simulink model "CrCtl_StTrans"  (R2016b)
settings: configuration reference "CodeGenConfigSet" (kept outside this file)
values from neighbouring files (symbols this model uses):
  CrCtl_swtAllwSetDrngOvrd_C = Calibration.Parameter    [init_CrCtl_StTrans.m]
  CrCtl_swtWESDem_C = Calibration.Parameter    [init_CrCtl_StTrans.m]
  CrCtl_tiEnaAftShOff_C = Calibration.Parameter    [init_CrCtl_StTrans.m]
  CrCtl_vAcclLoLim_C = Calibration.Parameter    [init_CrCtl_StTrans.m]
  CrCtl_vAcclUpLim_C = Calibration.Parameter    [init_CrCtl_StTrans.m]
  CrCtl_vDeclLoLim_C = Calibration.Parameter    [init_CrCtl_StTrans.m]
  CrCtl_vDeclUpLim_C = Calibration.Parameter    [init_CrCtl_StTrans.m]
  CrCtl_vEnaAftShOff_C = Calibration.Parameter    [init_CrCtl_StTrans.m]
  CrCtl_vMinAct_C = Calibration.Parameter    [init_CrCtl_StTrans.m]
  MoFCCtl_vCrCtlMin_C = Calibration.Parameter    [init_CrCtl_StTrans.m]
  VEL_ZERO = fi(0,VehSpeed_km_h)    [init_CrCtl_StTrans.m]
undefined symbols (not defined in the file or in its folder): CrCtl_stLck_conv, CrCtl_stOpFunc_conv, CrCtl_stShOff_conv, CrCtl_stSub_conv, CrCtl_StTrans_DT, CrCUI_BttnState_conv, CruiseCtl_State_conv, WESDem_State_conv
libraries: CXLib x4
settings Model: Creator=guanxiaoxing  LastModifiedBy=guanxiaoxing
settings ConfigSetRef: SourceLocation=Base Workspace

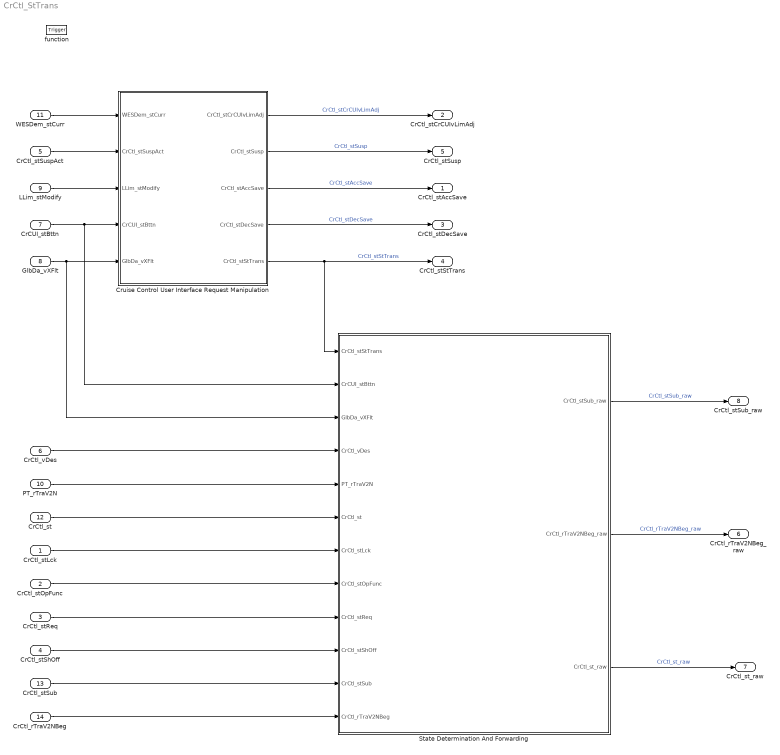
== system CrCtl_StTrans ==
  CrCtl_stLck : Inport  Description=Cruise Control lock Status  OutDataTypeStr=Enum: CrCtl_stLck_conv
  CrCtl_stOpFunc : Inport  Description=state of cruise control operation functionality  Port=2  OutDataTypeStr=Enum: CrCtl_stOpFunc_conv
  CrCtl_stReq : Inport  Description=Cruise control is active  Port=3  OutMin=0  OutMax=1  OutDataTypeStr=boolean
  CrCtl_stShOff : Inport  Description=cruise control shut-off requirement  Port=4  OutDataTypeStr=Enum: CrCtl_stShOff_conv
  CrCtl_stSuspAct : Inport  Description=Cruise Control suspend mode active Status  Port=5  OutMin=0  OutMax=1  OutDataTypeStr=boolean
  CrCtl_vDes : Inport  Tag=km/h  Description=Cruise Control desired set point speed  Port=6  OutMin=0  OutMax=250  OutDataTypeStr=VehSpeed_km_h
  CrCUI_stBttn : Inport  Description=Application parameter for status button information  Port=7  OutDataTypeStr=Enum: CrCUI_BttnState_conv
  GlbDa_vXFlt : Inport  Tag=km/h  Description=Vehicle velocity filtered  Port=8  OutMin=0  OutMax=250  OutDataTypeStr=VehSpeed_km_h
  LLim_stModify : Inport  Description=Application parameter for Status for changing adjustable vehicle speed limit  Port=9  OutMin=0  OutMax=1  OutDataTypeStr=boolean
  PT_rTraV2N : Inport  Tag=km/h/rpm  Description=Quotient of velocity and engine speed  Port=10  OutMin=-0.32768  OutMax=0.32767  OutDataTypeStr=Tra_V2N_km_h_rpm
  WESDem_stCurr : Inport  Description=Status of the working engine Speed Control  Port=11  OutDataTypeStr=Enum: WESDem_State_conv
  CrCtl_st : Inport  Description=Application parameter for Cruise Control state  Port=12  OutDataTypeStr=Enum: CruiseCtl_State_conv
  CrCtl_stSub : Inport  Description=Cruise control sub mode  Port=13  OutDataTypeStr=Enum: CrCtl_stSub_conv
  CrCtl_rTraV2NBeg : Inport  Tag=km/h/rpm  Description=V/N ratio at activation of cruise control  Port=14  OutMin=-0.32768  OutMax=0.32767  OutDataTypeStr=Tra_V2N_km_h_rpm
  function : TriggerPort  TriggerType=function-call  VariantControl=Variant
  Cruise Control User Interface Request Manipulation : Subsystem
  State Determination And Forwarding : Subsystem
  CrCtl_stAccSave : Outport  Description=|  OutDataTypeStr=Enum: CrCUI_BttnState_conv
      | Last CrCui state below the minimum speed to
      | activate
  CrCtl_stCrCUIvLimAdj : Outport  Description=CrCui Status of Limitation adjustment by Cruise control  Port=2  OutDataTypeStr=Enum: CrCUI_BttnState_conv
  CrCtl_stDecSave : Outport  Description=|  Port=3  OutDataTypeStr=Enum: CrCUI_BttnState_conv
      | Last CrCui state above the minimum speed to
      | activate
  CrCtl_stStTrans : Outport  Description=State transition demand to the state machine of cruise control  Port=4  OutDataTypeStr=Enum: CrCUI_BttnState_conv
  CrCtl_stSusp : Outport  Description=Status of Cruise control suspend mode  Port=5  OutDataTypeStr=Enum: CrCUI_BttnState_conv
  CrCtl_rTraV2NBeg_raw : Outport  Tag=km/h/rpm  Description=V/N ratio at activation of cruise control  Port=6  OutMin=-0.32768  OutMax=0.32767  OutDataTypeStr=Tra_V2N_km_h_rpm
  CrCtl_st_raw : Outport  Description=Application parameter for Cruise Control state  Port=7  OutDataTypeStr=Enum: CruiseCtl_State_conv
  CrCtl_stSub_raw : Outport  Description=Cruise control sub mode  Port=8  OutDataTypeStr=Enum: CrCtl_stSub_conv
  wires:
  WESDem_stCurr/1 -> Cruise Control User Interface Request Manipulation/1(WESDem_stCurr)
  CrCtl_stSuspAct/1 -> Cruise Control User Interface Request Manipulation/2(CrCtl_stSuspAct)
  LLim_stModify/1 -> Cruise Control User Interface Request Manipulation/3(LLim_stModify)
  CrCUI_stBttn/1 -> Cruise Control User Interface Request Manipulation/4(CrCUI_stBttn), State Determination And Forwarding/2(CrCUI_stBttn)
  GlbDa_vXFlt/1 -> Cruise Control User Interface Request Manipulation/5(GlbDa_vXFlt), State Determination And Forwarding/3(GlbDa_vXFlt)
  CrCtl_stShOff/1 -> State Determination And Forwarding/10(CrCtl_stShOff)
  CrCtl_stLck/1 -> State Determination And Forwarding/7(CrCtl_stLck)
  CrCtl_stReq/1 -> State Determination And Forwarding/9(CrCtl_stReq)
  PT_rTraV2N/1 -> State Determination And Forwarding/5(PT_rTraV2N)
  CrCtl_vDes/1 -> State Determination And Forwarding/4(CrCtl_vDes)
  CrCtl_stOpFunc/1 -> State Determination And Forwarding/8(CrCtl_stOpFunc)
  Cruise Control User Interface Request Manipulation/5(CrCtl_stStTrans) -> CrCtl_stStTrans/1, State Determination And Forwarding/1(CrCtl_stStTrans)  "CrCtl_stStTrans"
  Cruise Control User Interface Request Manipulation/1(CrCtl_stCrCUIvLimAdj) -> CrCtl_stCrCUIvLimAdj/1  "CrCtl_stCrCUIvLimAdj"
  Cruise Control User Interface Request Manipulation/3(CrCtl_stAccSave) -> CrCtl_stAccSave/1  "CrCtl_stAccSave"
  Cruise Control User Interface Request Manipulation/4(CrCtl_stDecSave) -> CrCtl_stDecSave/1  "CrCtl_stDecSave"
  Cruise Control User Interface Request Manipulation/2(CrCtl_stSusp) -> CrCtl_stSusp/1  "CrCtl_stSusp"
  State Determination And Forwarding/2(CrCtl_rTraV2NBeg_raw) -> CrCtl_rTraV2NBeg_raw/1  "CrCtl_rTraV2NBeg_raw"
  CrCtl_st/1 -> State Determination And Forwarding/6(CrCtl_st)
  State Determination And Forwarding/3(CrCtl_st_raw) -> CrCtl_st_raw/1  "CrCtl_st_raw"
  State Determination And Forwarding/1(CrCtl_stSub_raw) -> CrCtl_stSub_raw/1  "CrCtl_stSub_raw"
  CrCtl_stSub/1 -> State Determination And Forwarding/11(CrCtl_stSub)
  CrCtl_rTraV2NBeg/1 -> State Determination And Forwarding/12(CrCtl_rTraV2NBeg)

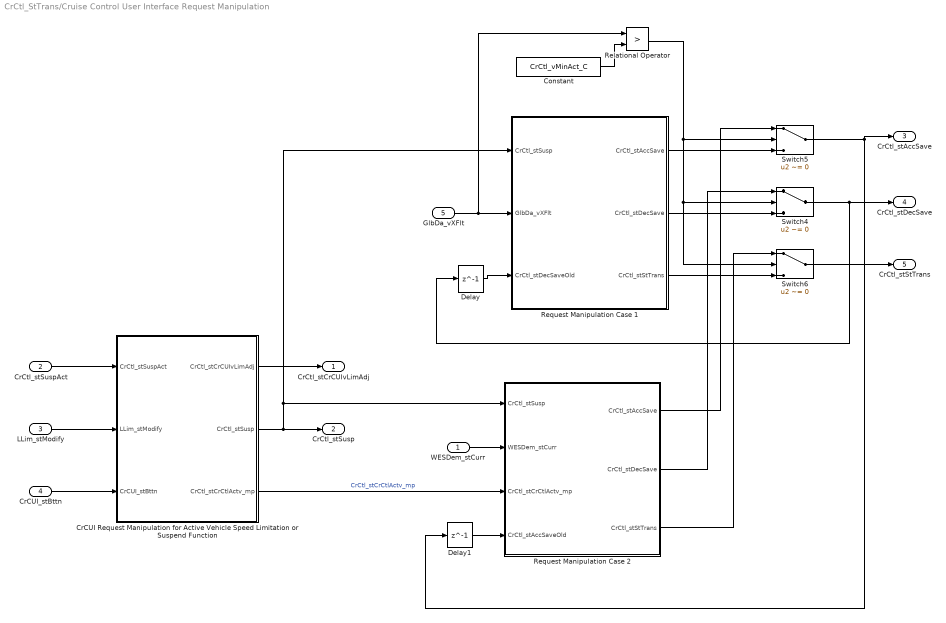
== system CrCtl_StTrans/Cruise Control User Interface Request Manipulation ==
  WESDem_stCurr : Inport
  CrCtl_stSuspAct : Inport  Port=2
  LLim_stModify : Inport  Port=3
  CrCUI_stBttn : Inport  Port=4
  GlbDa_vXFlt : Inport  Port=5
  Constant : Constant  Value=CrCtl_vMinAct_C
  CrCUI Request Manipulation for Active Vehicle Speed Limitation or Suspend Function : Subsystem
  Delay : Delay  DelayLength=1  InitialCondition=CrCUI_BttnState_conv.CRCUI_NEUTR  InputProcessing=Columns as channels (frame based)
  Delay1 : Delay  DelayLength=1  InitialCondition=CrCUI_BttnState_conv.CRCUI_NEUTR
  Relational Operator : RelationalOperator  Operator=>  OutDataTypeStr=boolean  RndMeth=Simplest
  Request Manipulation Case 1 : Subsystem
  Request Manipulation Case 2 : Subsystem
  Switch4 : Switch  Criteria=u2 ~= 0
  Switch5 : Switch  Criteria=u2 ~= 0
  Switch6 : Switch  Criteria=u2 ~= 0
  CrCtl_stCrCUIvLimAdj : Outport
  CrCtl_stSusp : Outport  Port=2
  CrCtl_stAccSave : Outport  Port=3
  CrCtl_stDecSave : Outport  Port=4
  CrCtl_stStTrans : Outport  Port=5
  wires:
  CrCUI Request Manipulation for Active Vehicle Speed Limitation or Suspend Function/2(CrCtl_stSusp) -> CrCtl_stSusp/1, Request Manipulation Case 1/1(CrCtl_stSusp), Request Manipulation Case 2/1(CrCtl_stSusp)
  WESDem_stCurr/1 -> Request Manipulation Case 2/2(WESDem_stCurr)
  Relational Operator/1 -> Switch6/2, Switch4/2, Switch5/2
  Request Manipulation Case 1/1(CrCtl_stAccSave) -> Switch5/3
  Request Manipulation Case 2/1(CrCtl_stAccSave) -> Switch5/1
  Request Manipulation Case 1/2(CrCtl_stDecSave) -> Switch4/3
  Request Manipulation Case 2/2(CrCtl_stDecSave) -> Switch4/1
  Request Manipulation Case 1/3(CrCtl_stStTrans) -> Switch6/3
  Request Manipulation Case 2/3(CrCtl_stStTrans) -> Switch6/1
  Switch5/1 -> CrCtl_stAccSave/1, Delay1/1
  Switch4/1 -> Delay/1, CrCtl_stDecSave/1
  Switch6/1 -> CrCtl_stStTrans/1
  CrCUI Request Manipulation for Active Vehicle Speed Limitation or Suspend Function/1(CrCtl_stCrCUIvLimAdj) -> CrCtl_stCrCUIvLimAdj/1
  CrCUI Request Manipulation for Active Vehicle Speed Limitation or Suspend Function/3(CrCtl_stCrCtlActv_mp) -> Request Manipulation Case 2/3(CrCtl_stCrCtlActv_mp)  "CrCtl_stCrCtlActv_mp"
  CrCtl_stSuspAct/1 -> CrCUI Request Manipulation for Active Vehicle Speed Limitation or Suspend Function/1(CrCtl_stSuspAct)
  LLim_stModify/1 -> CrCUI Request Manipulation for Active Vehicle Speed Limitation or Suspend Function/2(LLim_stModify)
  CrCUI_stBttn/1 -> CrCUI Request Manipulation for Active Vehicle Speed Limitation or Suspend Function/3(CrCUI_stBttn)
  GlbDa_vXFlt/1 -> Relational Operator/1, Request Manipulation Case 1/2(GlbDa_vXFlt)
  Constant/1 -> Relational Operator/2
  Delay/1 -> Request Manipulation Case 1/3(CrCtl_stDecSaveOld)
  Delay1/1 -> Request Manipulation Case 2/4(CrCtl_stAccSaveOld)

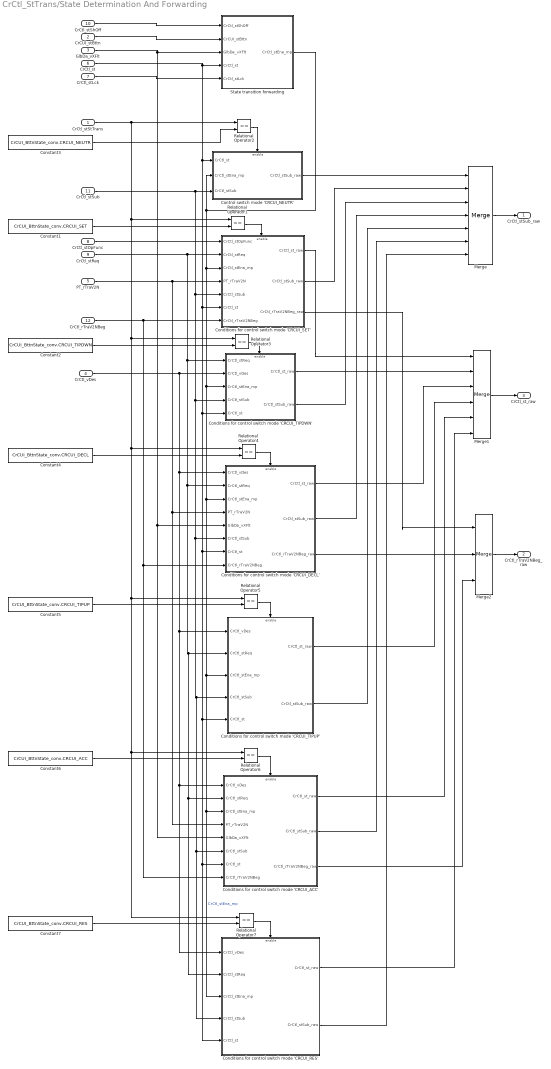
== system CrCtl_StTrans/State Determination And Forwarding ==
  CrCtl_stStTrans : Inport
  CrCUI_stBttn : Inport  Port=2
  GlbDa_vXFlt : Inport  Port=3
  CrCtl_vDes : Inport  Port=4
  PT_rTraV2N : Inport  Port=5
  CrCtl_st : Inport  Port=6
  CrCtl_stLck : Inport  Port=7
  CrCtl_stOpFunc : Inport  Port=8
  CrCtl_stReq : Inport  Port=9
  CrCtl_stShOff : Inport  Port=10
  CrCtl_stSub : Inport  Port=11
  CrCtl_rTraV2NBeg : Inport  Port=12
  "Conditions for control switch mode 'CRCUI_ACC' " : Subsystem
  Conditions for control switch mode 'CRCUI_DECL' : Subsystem
  Conditions for control switch mode 'CRCUI_RES' : Subsystem
  "Conditions for control switch mode 'CRCUI_SET' " : Subsystem
  Conditions for control switch mode 'CRCUI_TIPDWN' : Subsystem
  Conditions for control switch mode 'CRCUI_TIPUP' : Subsystem
  Constant1 : Constant  Value=CrCUI_BttnState_conv.CRCUI_SET
  Constant2 : Constant  Value=CrCUI_BttnState_conv.CRCUI_TIPDWN
  Constant3 : Constant  Value=CrCUI_BttnState_conv.CRCUI_NEUTR
  Constant4 : Constant  Value=CrCUI_BttnState_conv.CRCUI_DECL
  Constant5 : Constant  Value=CrCUI_BttnState_conv.CRCUI_TIPUP
  Constant6 : Constant  Value=CrCUI_BttnState_conv.CRCUI_ACC
  Constant7 : Constant  Value=CrCUI_BttnState_conv.CRCUI_RES
  Control switch mode 'CRCUI_NEUTR' : Subsystem
  Merge : Merge  Inputs=7
  Merge1 : Merge  Inputs=6
  Merge2 : Merge  Inputs=3
  Relational Operator{1..7} (7 alike) : RelationalOperator  Operator===  OutDataTypeStr=boolean  RndMeth=Simplest
  State transition forwarding : Subsystem
  CrCtl_stSub_raw : Outport
  CrCtl_rTraV2NBeg_raw : Outport  Port=2
  CrCtl_st_raw : Outport  Port=3
  wires:
  CrCtl_vDes/1 -> Conditions for control switch mode 'CRCUI_RES'/1(CrCtl_vDes), "Conditions for control switch mode 'CRCUI_ACC' "/1(CrCtl_vDes), Conditions for control switch mode 'CRCUI_TIPUP'/1(CrCtl_vDes), Conditions for control switch mode 'CRCUI_DECL'/1(CrCtl_vDes), Conditions for control switch mode 'CRCUI_TIPDWN'/2(CrCtl_vDes)
  PT_rTraV2N/1 -> "Conditions for control switch mode 'CRCUI_ACC' "/4(PT_rTraV2N), Conditions for control switch mode 'CRCUI_DECL'/4(PT_rTraV2N), "Conditions for control switch mode 'CRCUI_SET' "/4(PT_rTraV2N)
  CrCtl_stOpFunc/1 -> "Conditions for control switch mode 'CRCUI_SET' "/1(CrCtl_stOpFunc)
  CrCtl_stReq/1 -> Conditions for control switch mode 'CRCUI_RES'/2(CrCtl_stReq), "Conditions for control switch mode 'CRCUI_ACC' "/2(CrCtl_stReq), Conditions for control switch mode 'CRCUI_TIPUP'/2(CrCtl_stReq), Conditions for control switch mode 'CRCUI_DECL'/2(CrCtl_stReq), Conditions for control switch mode 'CRCUI_TIPDWN'/1(CrCtl_stReq), "Conditions for control switch mode 'CRCUI_SET' "/2(CrCtl_stReq)
  State transition forwarding/1(CrCtl_stEna_mp) -> Conditions for control switch mode 'CRCUI_RES'/3(CrCtl_stEna_mp), "Conditions for control switch mode 'CRCUI_ACC' "/3(CrCtl_stEna_mp), Conditions for control switch mode 'CRCUI_TIPUP'/3(CrCtl_stEna_mp), Conditions for control switch mode 'CRCUI_DECL'/3(CrCtl_stEna_mp), Conditions for control switch mode 'CRCUI_TIPDWN'/3(CrCtl_stEna_mp), "Conditions for control switch mode 'CRCUI_SET' "/3(CrCtl_stEna_mp), Control switch mode 'CRCUI_NEUTR'/2(CrCtl_stEna_mp)  "CrCtl_stEna_mp"
  CrCUI_stBttn/1 -> State transition forwarding/2(CrCUI_stBttn)
  GlbDa_vXFlt/1 -> "Conditions for control switch mode 'CRCUI_ACC' "/5(GlbDa_vXFlt), Conditions for control switch mode 'CRCUI_DECL'/5(GlbDa_vXFlt), State transition forwarding/3(GlbDa_vXFlt)
  CrCtl_stLck/1 -> State transition forwarding/5(CrCtl_stLck)
  CrCtl_stShOff/1 -> State transition forwarding/1(CrCtl_stShOff)
  Constant3/1 -> Relational Operator2/2
  Relational Operator2/1 -> Control switch mode 'CRCUI_NEUTR'/Enable
  Constant1/1 -> Relational Operator1/2
  Relational Operator1/1 -> "Conditions for control switch mode 'CRCUI_SET' "/Enable
  Constant2/1 -> Relational Operator3/2
  Relational Operator3/1 -> Conditions for control switch mode 'CRCUI_TIPDWN'/Enable
  Constant4/1 -> Relational Operator4/2
  Relational Operator4/1 -> Conditions for control switch mode 'CRCUI_DECL'/Enable
  Constant5/1 -> Relational Operator5/2
  Relational Operator5/1 -> Conditions for control switch mode 'CRCUI_TIPUP'/Enable
  Constant6/1 -> Relational Operator6/2
  Relational Operator6/1 -> "Conditions for control switch mode 'CRCUI_ACC' "/Enable
  Constant7/1 -> Relational Operator7/2
  CrCtl_stStTrans/1 -> Relational Operator2/1, Relational Operator7/1, Relational Operator6/1, Relational Operator5/1, Relational Operator4/1, Relational Operator3/1, Relational Operator1/1
  Relational Operator7/1 -> Conditions for control switch mode 'CRCUI_RES'/Enable
  Merge/1 -> CrCtl_stSub_raw/1
  Merge1/1 -> CrCtl_st_raw/1
  CrCtl_stSub/1 -> "Conditions for control switch mode 'CRCUI_SET' "/5(CrCtl_stSub), Conditions for control switch mode 'CRCUI_TIPDWN'/4(CrCtl_stSub), Conditions for control switch mode 'CRCUI_RES'/4(CrCtl_stSub), "Conditions for control switch mode 'CRCUI_ACC' "/6(CrCtl_stSub), Conditions for control switch mode 'CRCUI_TIPUP'/4(CrCtl_stSub), Conditions for control switch mode 'CRCUI_DECL'/6(CrCtl_stSub), Control switch mode 'CRCUI_NEUTR'/3(CrCtl_stSub)
  Merge2/1 -> CrCtl_rTraV2NBeg_raw/1
  CrCtl_rTraV2NBeg/1 -> "Conditions for control switch mode 'CRCUI_ACC' "/8(CrCtl_rTraV2NBeg), Conditions for control switch mode 'CRCUI_DECL'/8(CrCtl_rTraV2NBeg), "Conditions for control switch mode 'CRCUI_SET' "/7(CrCtl_rTraV2NBeg)
  CrCtl_st/1 -> Conditions for control switch mode 'CRCUI_RES'/5(CrCtl_st), "Conditions for control switch mode 'CRCUI_ACC' "/7(CrCtl_st), Conditions for control switch mode 'CRCUI_TIPUP'/5(CrCtl_st), Conditions for control switch mode 'CRCUI_DECL'/7(CrCtl_st), Conditions for control switch mode 'CRCUI_TIPDWN'/5(CrCtl_st), "Conditions for control switch mode 'CRCUI_SET' "/6(CrCtl_st), Control switch mode 'CRCUI_NEUTR'/1(CrCtl_st), State transition forwarding/4(CrCtl_st)
  Control switch mode 'CRCUI_NEUTR'/1(CrCtl_stSub_raw) -> Merge/1
  "Conditions for control switch mode 'CRCUI_SET' "/1(CrCtl_st_raw) -> Merge1/1
  "Conditions for control switch mode 'CRCUI_SET' "/2(CrCtl_stSub_raw) -> Merge/2
  "Conditions for control switch mode 'CRCUI_SET' "/3(CrCtl_rTraV2NBeg_raw) -> Merge2/1
  Conditions for control switch mode 'CRCUI_TIPDWN'/1(CrCtl_st_raw) -> Merge1/2
  Conditions for control switch mode 'CRCUI_TIPDWN'/2(CrCtl_stSub_raw) -> Merge/3
  Conditions for control switch mode 'CRCUI_DECL'/1(CrCtl_st_raw) -> Merge1/3
  Conditions for control switch mode 'CRCUI_DECL'/2(CrCtl_stSub_raw) -> Merge/4
  Conditions for control switch mode 'CRCUI_TIPUP'/1(CrCtl_st_raw) -> Merge1/4
  Conditions for control switch mode 'CRCUI_TIPUP'/2(CrCtl_stSub_raw) -> Merge/5
  "Conditions for control switch mode 'CRCUI_ACC' "/1(CrCtl_st_raw) -> Merge1/5
  "Conditions for control switch mode 'CRCUI_ACC' "/2(CrCtl_stSub_raw) -> Merge/6
  Conditions for control switch mode 'CRCUI_RES'/1(CrCtl_st_raw) -> Merge1/6
  Conditions for control switch mode 'CRCUI_RES'/2(CrCtl_stSub_raw) -> Merge/7
  "Conditions for control switch mode 'CRCUI_ACC' "/3(CrCtl_rTraV2NBeg_raw) -> Merge2/3
  Conditions for control switch mode 'CRCUI_DECL'/3(CrCtl_rTraV2NBeg_raw) -> Merge2/2

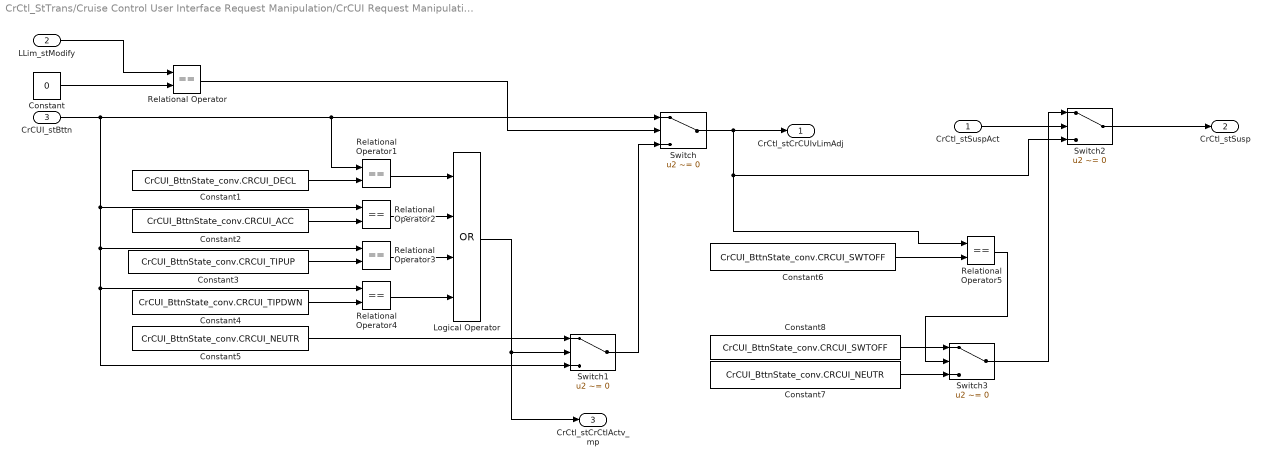
== system CrCtl_StTrans/Cruise Control User Interface Request Manipulation/CrCUI Request Manipulation for Active Vehicle Speed Limitation or Suspend Function ==
  CrCtl_stSuspAct : Inport
  LLim_stModify : Inport  Port=2
  CrCUI_stBttn : Inport  Port=3
  Constant : Constant  Value=0
  Constant1 : Constant  Value=CrCUI_BttnState_conv.CRCUI_DECL  VectorParams1D=off
  Constant2 : Constant  Value=CrCUI_BttnState_conv.CRCUI_ACC
  Constant3 : Constant  Value=CrCUI_BttnState_conv.CRCUI_TIPUP
  Constant4 : Constant  Value=CrCUI_BttnState_conv.CRCUI_TIPDWN
  Constant5 : Constant  Value=CrCUI_BttnState_conv.CRCUI_NEUTR
  Constant6 : Constant  Value=CrCUI_BttnState_conv.CRCUI_SWTOFF
  Constant7 : Constant  Value=CrCUI_BttnState_conv.CRCUI_NEUTR
  Constant8 : Constant  Value=CrCUI_BttnState_conv.CRCUI_SWTOFF
  Logical Operator : Logic  Operator=OR  Inputs=4  AllPortsSameDT=off  OutDataTypeStr=boolean
  Relational Operator{,1..5} (6 alike) : RelationalOperator  Operator===  OutDataTypeStr=boolean  RndMeth=Simplest
  Switch{,1..3} (4 alike) : Switch  Criteria=u2 ~= 0
  CrCtl_stCrCUIvLimAdj : Outport
  CrCtl_stSusp : Outport  Port=2
  CrCtl_stCrCtlActv_mp : Outport  Port=3
  wires:
  LLim_stModify/1 -> Relational Operator/1
  Constant/1 -> Relational Operator/2
  Relational Operator/1 -> Switch/2
  Constant1/1 -> Relational Operator1/2
  Constant3/1 -> Relational Operator3/2
  Constant7/1 -> Switch3/3
  Constant2/1 -> Relational Operator2/2
  Constant8/1 -> Switch3/1
  Switch/1 -> Switch2/3, Relational Operator5/1, CrCtl_stCrCUIvLimAdj/1
  Switch3/1 -> Switch2/1
  Relational Operator4/1 -> Logical Operator/4
  CrCtl_stSuspAct/1 -> Switch2/2
  Constant4/1 -> Relational Operator4/2
  CrCUI_stBttn/1 -> Switch/1, Relational Operator1/1, Switch1/3, Relational Operator4/1, Relational Operator3/1, Relational Operator2/1
  Relational Operator1/1 -> Logical Operator/1
  Relational Operator2/1 -> Logical Operator/2
  Relational Operator5/1 -> Switch3/2
  Logical Operator/1 -> CrCtl_stCrCtlActv_mp/1, Switch1/2
  Relational Operator3/1 -> Logical Operator/3
  Constant6/1 -> Relational Operator5/2
  Switch1/1 -> Switch/3
  Constant5/1 -> Switch1/1
  Switch2/1 -> CrCtl_stSusp/1

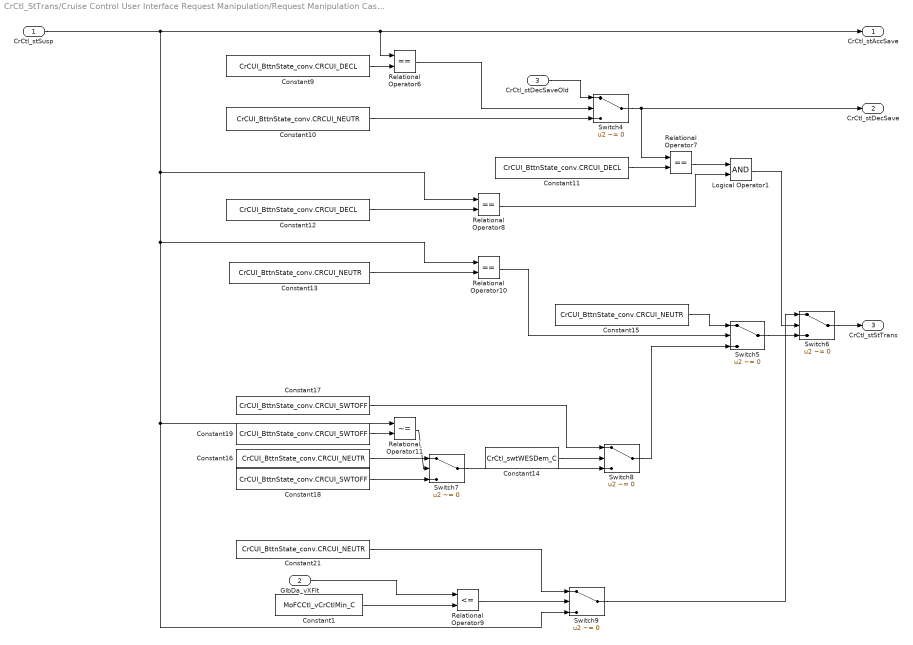
== system CrCtl_StTrans/Cruise Control User Interface Request Manipulation/Request Manipulation Case 1 ==
  CrCtl_stSusp : Inport
  GlbDa_vXFlt : Inport  Port=2
  CrCtl_stDecSaveOld : Inport  Port=3
  Constant1 : Constant  Value=MoFCCtl_vCrCtlMin_C
  Constant{10,13,15..16,21} (5 alike) : Constant  Value=CrCUI_BttnState_conv.CRCUI_NEUTR
  Constant11 : Constant  Value=CrCUI_BttnState_conv.CRCUI_DECL
  Constant12 : Constant  Value=CrCUI_BttnState_conv.CRCUI_DECL
  Constant14 : Constant  Value=CrCtl_swtWESDem_C
  Constant17 : Constant  Value=CrCUI_BttnState_conv.CRCUI_SWTOFF
  Constant18 : Constant  Value=CrCUI_BttnState_conv.CRCUI_SWTOFF
  Constant19 : Constant  Value=CrCUI_BttnState_conv.CRCUI_SWTOFF
  Constant9 : Constant  Value=CrCUI_BttnState_conv.CRCUI_DECL
  Logical Operator1 : Logic  AllPortsSameDT=off  OutDataTypeStr=boolean
  Relational Operator{6..8,10} (4 alike) : RelationalOperator  Operator===  OutDataTypeStr=boolean  RndMeth=Simplest
  Relational Operator11 : RelationalOperator  Operator=~=  OutDataTypeStr=boolean  RndMeth=Simplest
  Relational Operator9 : RelationalOperator  Operator=<=  OutDataTypeStr=boolean  RndMeth=Simplest
  Switch{4..9} (6 alike) : Switch  Criteria=u2 ~= 0
  CrCtl_stAccSave : Outport
  CrCtl_stDecSave : Outport  Port=2
  CrCtl_stStTrans : Outport  Port=3
  wires:
  Constant9/1 -> Relational Operator6/2
  Relational Operator8/1 -> Logical Operator1/2
  Constant15/1 -> Switch5/1
  Relational Operator6/1 -> Switch4/2
  Constant10/1 -> Switch4/3
  Switch4/1 -> Relational Operator7/1, CrCtl_stDecSave/1
  GlbDa_vXFlt/1 -> Relational Operator9/1
  Switch7/1 -> Switch8/3
  Switch5/1 -> Switch6/3
  Constant17/1 -> Switch8/1
  Constant1/1 -> Relational Operator9/2
  Switch6/1 -> CrCtl_stStTrans/1
  Relational Operator7/1 -> Logical Operator1/1
  Constant18/1 -> Switch7/3
  Constant13/1 -> Relational Operator10/2
  Constant16/1 -> Switch7/1
  CrCtl_stSusp/1 -> CrCtl_stAccSave/1, Relational Operator6/1, Relational Operator8/1, Relational Operator10/1, Switch9/3, Relational Operator11/1
  Constant19/1 -> Relational Operator11/2
  Switch8/1 -> Switch5/3
  Relational Operator9/1 -> Switch9/2
  Constant14/1 -> Switch8/2
  Constant21/1 -> Switch9/1
  Logical Operator1/1 -> Switch6/2
  Constant12/1 -> Relational Operator8/2
  Relational Operator10/1 -> Switch5/2
  Constant11/1 -> Relational Operator7/2
  Relational Operator11/1 -> Switch7/2
  Switch9/1 -> Switch6/1
  CrCtl_stDecSaveOld/1 -> Switch4/1

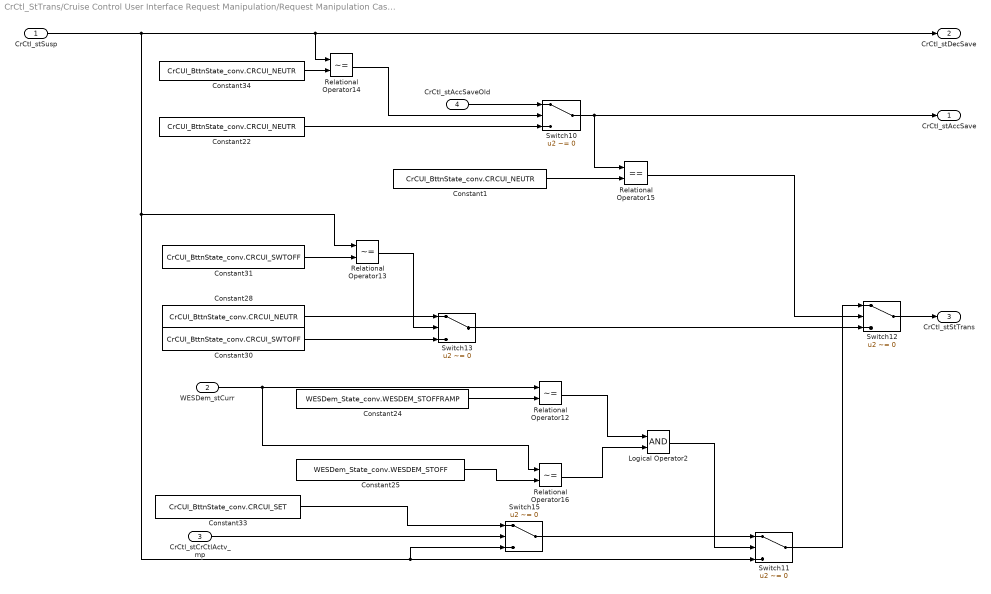
== system CrCtl_StTrans/Cruise Control User Interface Request Manipulation/Request Manipulation Case 2 ==
  CrCtl_stSusp : Inport
  WESDem_stCurr : Inport  Port=2
  CrCtl_stCrCtlActv_mp : Inport  Port=3
  CrCtl_stAccSaveOld : Inport  Port=4
  Constant{1,22,28,34} (4 alike) : Constant  Value=CrCUI_BttnState_conv.CRCUI_NEUTR
  Constant24 : Constant  Value=WESDem_State_conv.WESDEM_STOFFRAMP
  Constant25 : Constant  Value=WESDem_State_conv.WESDEM_STOFF
  Constant30 : Constant  Value=CrCUI_BttnState_conv.CRCUI_SWTOFF
  Constant31 : Constant  Value=CrCUI_BttnState_conv.CRCUI_SWTOFF
  Constant33 : Constant  Value=CrCUI_BttnState_conv.CRCUI_SET
  Logical Operator2 : Logic  AllPortsSameDT=off  OutDataTypeStr=boolean
  Relational Operator{12..14,16} (4 alike) : RelationalOperator  Operator=~=  OutDataTypeStr=boolean  RndMeth=Simplest
  Relational Operator15 : RelationalOperator  Operator===  OutDataTypeStr=boolean  RndMeth=Simplest
  Switch{10..13,15} (5 alike) : Switch  Criteria=u2 ~= 0
  CrCtl_stAccSave : Outport
  CrCtl_stDecSave : Outport  Port=2
  CrCtl_stStTrans : Outport  Port=3
  wires:
  CrCtl_stCrCtlActv_mp/1 -> Switch15/2
  Constant25/1 -> Relational Operator16/2
  Constant34/1 -> Relational Operator14/2
  Relational Operator13/1 -> Switch13/2
  Relational Operator15/1 -> Switch12/2
  Relational Operator14/1 -> Switch10/2
  Constant28/1 -> Switch13/1
  Constant22/1 -> Switch10/3
  Constant33/1 -> Switch15/1
  Switch11/1 -> Switch12/1
  Constant1/1 -> Relational Operator15/2
  Switch13/1 -> Switch12/3
  Constant31/1 -> Relational Operator13/2
  Constant30/1 -> Switch13/3
  Relational Operator12/1 -> Logical Operator2/1
  Relational Operator16/1 -> Logical Operator2/2
  Switch15/1 -> Switch11/1
  Logical Operator2/1 -> Switch11/2
  Switch10/1 -> Relational Operator15/1, CrCtl_stAccSave/1
  CrCtl_stSusp/1 -> CrCtl_stDecSave/1, Relational Operator14/1, Relational Operator13/1, Switch11/3, Switch15/3
  Switch12/1 -> CrCtl_stStTrans/1
  Constant24/1 -> Relational Operator12/2
  WESDem_stCurr/1 -> Relational Operator12/1, Relational Operator16/1
  CrCtl_stAccSaveOld/1 -> Switch10/1

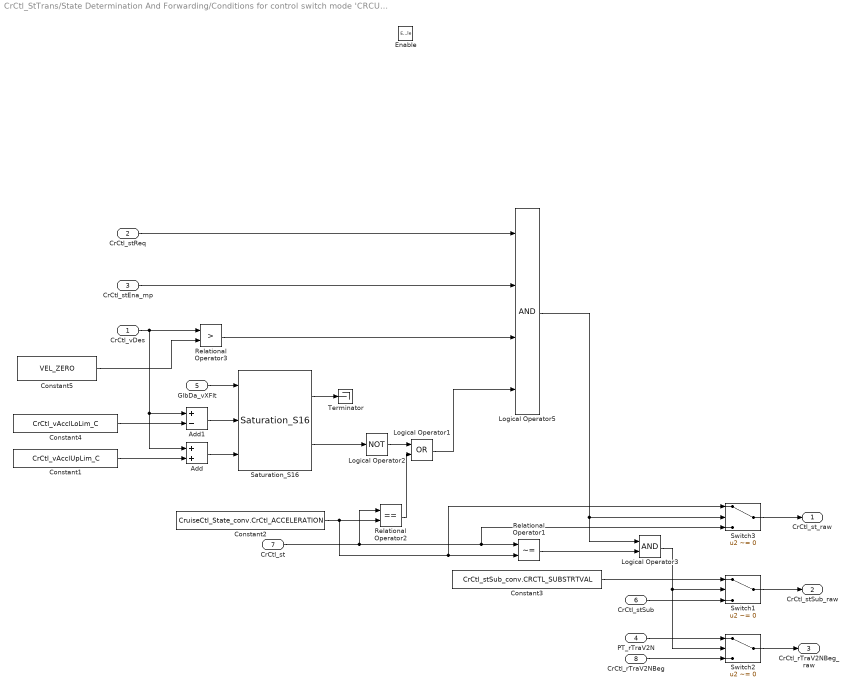
== system CrCtl_StTrans/State Determination And Forwarding/Conditions for control switch mode 'CRCUI_ACC'  ==
  CrCtl_vDes : Inport
  CrCtl_stReq : Inport  Port=2
  CrCtl_stEna_mp : Inport  Port=3
  PT_rTraV2N : Inport  Port=4
  GlbDa_vXFlt : Inport  Port=5
  CrCtl_stSub : Inport  Port=6
  CrCtl_st : Inport  Port=7
  CrCtl_rTraV2NBeg : Inport  Port=8
  Enable : EnablePort
  Add : Sum
  Add1 : Sum  Inputs=+-
  Constant1 : Constant  Value=CrCtl_vAcclUpLim_C
  Constant2 : Constant  Value=CruiseCtl_State_conv.CrCtl_ACCELERATION
  Constant3 : Constant  Value=CrCtl_stSub_conv.CRCTL_SUBSTRTVAL
  Constant4 : Constant  Value=CrCtl_vAcclLoLim_C
  Constant5 : Constant  Value=VEL_ZERO
  Logical Operator1 : Logic  Operator=OR  AllPortsSameDT=off  OutDataTypeStr=boolean
  Logical Operator2 : Logic  Operator=NOT  AllPortsSameDT=off  OutDataTypeStr=boolean
  Logical Operator3 : Logic  AllPortsSameDT=off  OutDataTypeStr=boolean
  Logical Operator5 : Logic  Inputs=4  AllPortsSameDT=off  OutDataTypeStr=boolean
  Relational Operator1 : RelationalOperator  Operator=~=  OutDataTypeStr=boolean  RndMeth=Simplest
  Relational Operator2 : RelationalOperator  Operator===  OutDataTypeStr=boolean  RndMeth=Simplest
  Relational Operator3 : RelationalOperator  Operator=>  OutDataTypeStr=boolean  RndMeth=Simplest
  Saturation_S16 : CXLib/Saturation_S16
  Switch1 : Switch  Criteria=u2 ~= 0
  Switch2 : Switch  Criteria=u2 ~= 0
  Switch3 : Switch  Criteria=u2 ~= 0
  Terminator : Terminator
  CrCtl_st_raw : Outport
  CrCtl_stSub_raw : Outport  Port=2
  CrCtl_rTraV2NBeg_raw : Outport  Port=3
  wires:
  Switch1/1 -> CrCtl_stSub_raw/1
  Constant3/1 -> Switch1/1
  CrCtl_st/1 -> Switch3/3, Relational Operator1/1, Relational Operator2/1
  PT_rTraV2N/1 -> Switch2/1
  Switch2/1 -> CrCtl_rTraV2NBeg_raw/1
  Switch3/1 -> CrCtl_st_raw/1
  CrCtl_stReq/1 -> Logical Operator5/1
  CrCtl_stEna_mp/1 -> Logical Operator5/2
  Constant5/1 -> Relational Operator3/2
  CrCtl_vDes/1 -> Relational Operator3/1, Add/1, Add1/1
  Relational Operator3/1 -> Logical Operator5/3
  Constant1/1 -> Add/2
  Constant4/1 -> Add1/2
  Constant2/1 -> Relational Operator2/2, Switch3/1, Relational Operator1/2
  Relational Operator1/1 -> Logical Operator3/2
  Logical Operator3/1 -> Switch2/2, Switch1/2
  Logical Operator5/1 -> Switch3/2, Logical Operator3/1
  Relational Operator2/1 -> Logical Operator1/2
  Logical Operator1/1 -> Logical Operator5/4
  Add1/1 -> Saturation_S16/2
  Add/1 -> Saturation_S16/3
  Logical Operator2/1 -> Logical Operator1/1
  CrCtl_stSub/1 -> Switch1/3
  CrCtl_rTraV2NBeg/1 -> Switch2/3
  Saturation_S16/1 -> Terminator/1
  Saturation_S16/2 -> Logical Operator2/1
  GlbDa_vXFlt/1 -> Saturation_S16/1

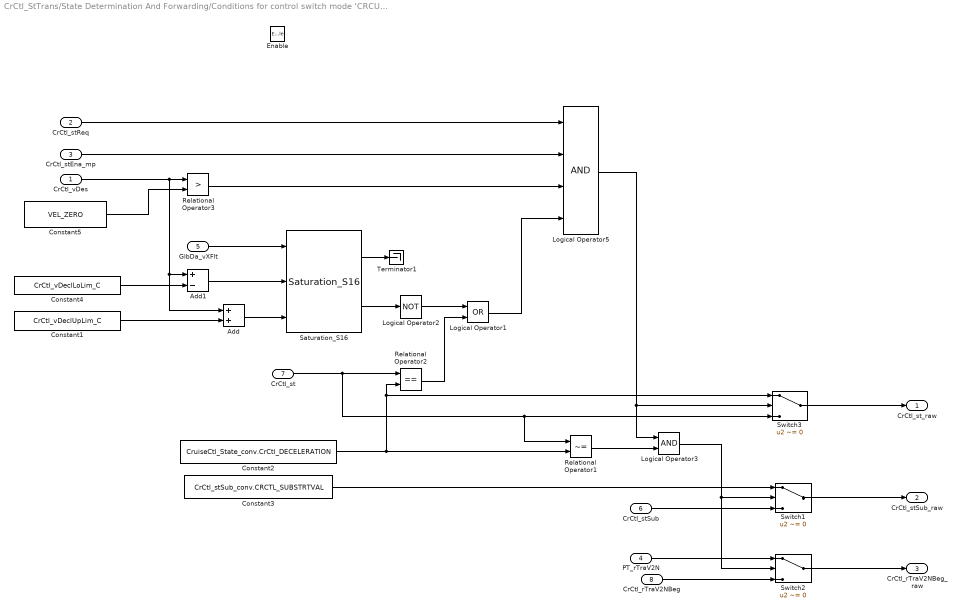
== system CrCtl_StTrans/State Determination And Forwarding/Conditions for control switch mode 'CRCUI_DECL' ==
  CrCtl_vDes : Inport
  CrCtl_stReq : Inport  Port=2
  CrCtl_stEna_mp : Inport  Port=3
  PT_rTraV2N : Inport  Port=4
  GlbDa_vXFlt : Inport  Port=5
  CrCtl_stSub : Inport  Port=6
  CrCtl_st : Inport  Port=7
  CrCtl_rTraV2NBeg : Inport  Port=8
  Enable : EnablePort
  Add : Sum
  Add1 : Sum  Inputs=+-
  Constant1 : Constant  Value=CrCtl_vDeclUpLim_C
  Constant2 : Constant  Value=CruiseCtl_State_conv.CrCtl_DECELERATION
  Constant3 : Constant  Value=CrCtl_stSub_conv.CRCTL_SUBSTRTVAL
  Constant4 : Constant  Value=CrCtl_vDeclLoLim_C
  Constant5 : Constant  Value=VEL_ZERO
  Logical Operator1 : Logic  Operator=OR  AllPortsSameDT=off  OutDataTypeStr=boolean
  Logical Operator2 : Logic  Operator=NOT  AllPortsSameDT=off  OutDataTypeStr=boolean
  Logical Operator3 : Logic  AllPortsSameDT=off  OutDataTypeStr=boolean
  Logical Operator5 : Logic  Inputs=4  AllPortsSameDT=off  OutDataTypeStr=boolean
  Relational Operator1 : RelationalOperator  Operator=~=  OutDataTypeStr=boolean  RndMeth=Simplest
  Relational Operator2 : RelationalOperator  Operator===  OutDataTypeStr=boolean  RndMeth=Simplest
  Relational Operator3 : RelationalOperator  Operator=>  OutDataTypeStr=boolean  RndMeth=Simplest
  Saturation_S16 : CXLib/Saturation_S16
  Switch1 : Switch  Criteria=u2 ~= 0
  Switch2 : Switch  Criteria=u2 ~= 0
  Switch3 : Switch  Criteria=u2 ~= 0
  Terminator1 : Terminator
  CrCtl_st_raw : Outport
  CrCtl_stSub_raw : Outport  Port=2
  CrCtl_rTraV2NBeg_raw : Outport  Port=3
  wires:
  Switch1/1 -> CrCtl_stSub_raw/1
  Constant3/1 -> Switch1/1
  PT_rTraV2N/1 -> Switch2/1
  Switch2/1 -> CrCtl_rTraV2NBeg_raw/1
  Switch3/1 -> CrCtl_st_raw/1
  CrCtl_stReq/1 -> Logical Operator5/1
  CrCtl_stEna_mp/1 -> Logical Operator5/2
  Constant5/1 -> Relational Operator3/2
  CrCtl_vDes/1 -> Add/1, Add1/1, Relational Operator3/1
  Relational Operator3/1 -> Logical Operator5/3
  Constant1/1 -> Add/2
  Constant4/1 -> Add1/2
  Constant2/1 -> Relational Operator1/2, Switch3/1, Relational Operator2/2
  Relational Operator1/1 -> Logical Operator3/2
  Logical Operator3/1 -> Switch2/2, Switch1/2
  Logical Operator5/1 -> Switch3/2, Logical Operator3/1
  Relational Operator2/1 -> Logical Operator1/2
  Logical Operator1/1 -> Logical Operator5/4
  GlbDa_vXFlt/1 -> Saturation_S16/1
  Logical Operator2/1 -> Logical Operator1/1
  CrCtl_st/1 -> Switch3/3, Relational Operator1/1, Relational Operator2/1
  Saturation_S16/1 -> Terminator1/1
  Add/1 -> Saturation_S16/3
  Add1/1 -> Saturation_S16/2
  Saturation_S16/2 -> Logical Operator2/1
  CrCtl_stSub/1 -> Switch1/3
  CrCtl_rTraV2NBeg/1 -> Switch2/3

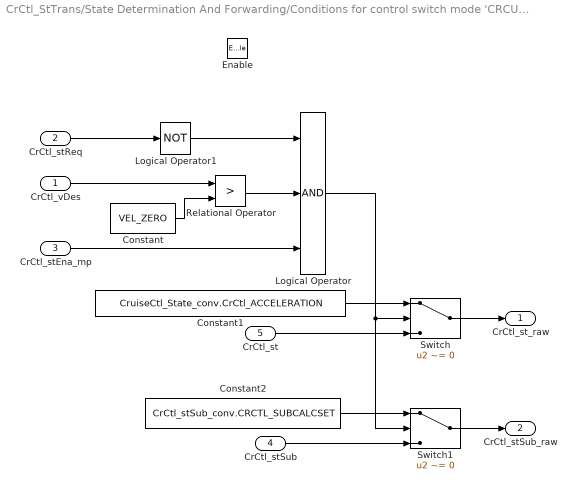
== system CrCtl_StTrans/State Determination And Forwarding/Conditions for control switch mode 'CRCUI_RES' ==
  CrCtl_vDes : Inport
  CrCtl_stReq : Inport  Port=2
  CrCtl_stEna_mp : Inport  Port=3
  CrCtl_stSub : Inport  Port=4
  CrCtl_st : Inport  Port=5
  Enable : EnablePort
  Constant : Constant  Value=VEL_ZERO
  Constant1 : Constant  Value=CruiseCtl_State_conv.CrCtl_ACCELERATION
  Constant2 : Constant  Value=CrCtl_stSub_conv.CRCTL_SUBCALCSET
  Logical Operator : Logic  Inputs=3  AllPortsSameDT=off  OutDataTypeStr=boolean
  Logical Operator1 : Logic  Operator=NOT  AllPortsSameDT=off  OutDataTypeStr=boolean
  Relational Operator : RelationalOperator  Operator=>  OutDataTypeStr=boolean  RndMeth=Simplest
  Switch : Switch  Criteria=u2 ~= 0
  Switch1 : Switch  Criteria=u2 ~= 0
  CrCtl_st_raw : Outport
  CrCtl_stSub_raw : Outport  Port=2
  wires:
  Switch1/1 -> CrCtl_stSub_raw/1
  Constant2/1 -> Switch1/1
  Constant1/1 -> Switch/1
  Switch/1 -> CrCtl_st_raw/1
  Relational Operator/1 -> Logical Operator/2
  CrCtl_stReq/1 -> Logical Operator1/1
  Constant/1 -> Relational Operator/2
  CrCtl_stEna_mp/1 -> Logical Operator/3
  CrCtl_vDes/1 -> Relational Operator/1
  Logical Operator/1 -> Switch1/2, Switch/2
  Logical Operator1/1 -> Logical Operator/1
  CrCtl_st/1 -> Switch/3
  CrCtl_stSub/1 -> Switch1/3

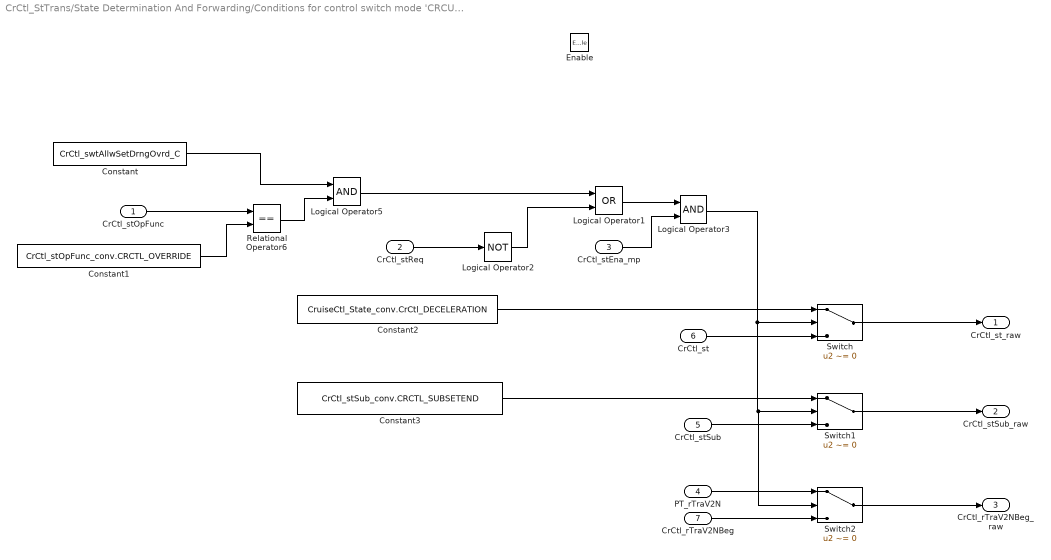
== system CrCtl_StTrans/State Determination And Forwarding/Conditions for control switch mode 'CRCUI_SET'  ==
  CrCtl_stOpFunc : Inport
  CrCtl_stReq : Inport  Port=2
  CrCtl_stEna_mp : Inport  Port=3
  PT_rTraV2N : Inport  Port=4
  CrCtl_stSub : Inport  Port=5
  CrCtl_st : Inport  Port=6
  CrCtl_rTraV2NBeg : Inport  Port=7
  Enable : EnablePort
  Constant : Constant  Value=CrCtl_swtAllwSetDrngOvrd_C
  Constant1 : Constant  Value=CrCtl_stOpFunc_conv.CRCTL_OVERRIDE
  Constant2 : Constant  Value=CruiseCtl_State_conv.CrCtl_DECELERATION
  Constant3 : Constant  Value=CrCtl_stSub_conv.CRCTL_SUBSETEND
  Logical Operator1 : Logic  Operator=OR  AllPortsSameDT=off  OutDataTypeStr=boolean
  Logical Operator2 : Logic  Operator=NOT  AllPortsSameDT=off  OutDataTypeStr=boolean
  Logical Operator3 : Logic  AllPortsSameDT=off  OutDataTypeStr=boolean
  Logical Operator5 : Logic  AllPortsSameDT=off  OutDataTypeStr=boolean
  Relational Operator6 : RelationalOperator  Operator===  OutDataTypeStr=boolean  RndMeth=Simplest
  Switch : Switch  Criteria=u2 ~= 0
  Switch1 : Switch  Criteria=u2 ~= 0
  Switch2 : Switch  Criteria=u2 ~= 0
  CrCtl_st_raw : Outport
  CrCtl_stSub_raw : Outport  Port=2
  CrCtl_rTraV2NBeg_raw : Outport  Port=3
  wires:
  Constant1/1 -> Relational Operator6/2
  Switch1/1 -> CrCtl_stSub_raw/1
  Constant3/1 -> Switch1/1
  Constant/1 -> Logical Operator5/1
  PT_rTraV2N/1 -> Switch2/1
  Logical Operator3/1 -> Switch2/2, Switch1/2, Switch/2
  Switch2/1 -> CrCtl_rTraV2NBeg_raw/1
  CrCtl_stReq/1 -> Logical Operator2/1
  CrCtl_stEna_mp/1 -> Logical Operator3/2
  Logical Operator2/1 -> Logical Operator1/2
  Switch/1 -> CrCtl_st_raw/1
  Logical Operator1/1 -> Logical Operator3/1
  Relational Operator6/1 -> Logical Operator5/2
  Constant2/1 -> Switch/1
  CrCtl_stOpFunc/1 -> Relational Operator6/1
  Logical Operator5/1 -> Logical Operator1/1
  CrCtl_st/1 -> Switch/3
  CrCtl_stSub/1 -> Switch1/3
  CrCtl_rTraV2NBeg/1 -> Switch2/3

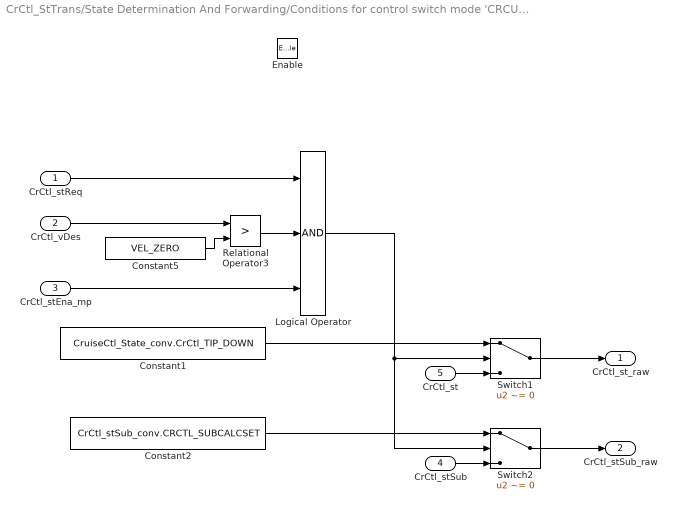
== system CrCtl_StTrans/State Determination And Forwarding/Conditions for control switch mode 'CRCUI_TIPDWN' ==
  CrCtl_stReq : Inport
  CrCtl_vDes : Inport  Port=2
  CrCtl_stEna_mp : Inport  Port=3
  CrCtl_stSub : Inport  Port=4
  CrCtl_st : Inport  Port=5
  Enable : EnablePort
  Constant1 : Constant  Value=CruiseCtl_State_conv.CrCtl_TIP_DOWN
  Constant2 : Constant  Value=CrCtl_stSub_conv.CRCTL_SUBCALCSET
  Constant5 : Constant  Value=VEL_ZERO
  Logical Operator : Logic  Inputs=3  AllPortsSameDT=off  OutDataTypeStr=boolean
  Relational Operator3 : RelationalOperator  Operator=>  OutDataTypeStr=boolean  RndMeth=Simplest
  Switch1 : Switch  Criteria=u2 ~= 0
  Switch2 : Switch  Criteria=u2 ~= 0
  CrCtl_st_raw : Outport
  CrCtl_stSub_raw : Outport  Port=2
  wires:
  CrCtl_stEna_mp/1 -> Logical Operator/3
  Relational Operator3/1 -> Logical Operator/2
  Constant5/1 -> Relational Operator3/2
  CrCtl_vDes/1 -> Relational Operator3/1
  Constant1/1 -> Switch1/1
  Switch1/1 -> CrCtl_st_raw/1
  Logical Operator/1 -> Switch2/2, Switch1/2
  Switch2/1 -> CrCtl_stSub_raw/1
  Constant2/1 -> Switch2/1
  CrCtl_stReq/1 -> Logical Operator/1
  CrCtl_st/1 -> Switch1/3
  CrCtl_stSub/1 -> Switch2/3

== system CrCtl_StTrans/State Determination And Forwarding/Conditions for control switch mode 'CRCUI_TIPUP' ==
  CrCtl_vDes : Inport
  CrCtl_stReq : Inport  Port=2
  CrCtl_stEna_mp : Inport  Port=3
  CrCtl_stSub : Inport  Port=4
  CrCtl_st : Inport  Port=5
  Enable : EnablePort
  Constant : Constant  Value=VEL_ZERO
  Constant1 : Constant  Value=CruiseCtl_State_conv.CrCtl_TIP_UP
  Constant2 : Constant  Value=CrCtl_stSub_conv.CRCTL_SUBCALCSET
  Logical Operator : Logic  Inputs=3  AllPortsSameDT=off  OutDataTypeStr=boolean
  Relational Operator : RelationalOperator  Operator=>  OutDataTypeStr=boolean  RndMeth=Simplest
  Switch : Switch  Criteria=u2 ~= 0
  Switch1 : Switch  Criteria=u2 ~= 0
  CrCtl_st_raw : Outport
  CrCtl_stSub_raw : Outport  Port=2
  wires:
  Switch1/1 -> CrCtl_stSub_raw/1
  Constant2/1 -> Switch1/1
  Constant1/1 -> Switch/1
  Switch/1 -> CrCtl_st_raw/1
  Relational Operator/1 -> Logical Operator/2
  CrCtl_stReq/1 -> Logical Operator/1
  Constant/1 -> Relational Operator/2
  CrCtl_stEna_mp/1 -> Logical Operator/3
  CrCtl_vDes/1 -> Relational Operator/1
  Logical Operator/1 -> Switch1/2, Switch/2
  CrCtl_st/1 -> Switch/3
  CrCtl_stSub/1 -> Switch1/3

== system CrCtl_StTrans/State Determination And Forwarding/Control switch mode 'CRCUI_NEUTR' ==
  CrCtl_st : Inport
  CrCtl_stEna_mp : Inport  Port=2
  CrCtl_stSub : Inport  Port=3
  Enable : EnablePort
  Constant10 : Constant  Value=CrCtl_stSub_conv.CRCTL_SUBRMPEND
  Constant7 : Constant  Value=CruiseCtl_State_conv.CrCtl_DECELERATION
  Constant8 : Constant  Value=CruiseCtl_State_conv.CrCtl_ACCELERATION
  Constant9 : Constant  Value=CrCtl_stSub_conv.CRCTL_SUBRMP
  Logical Operator4 : Logic  Inputs=3  AllPortsSameDT=off  OutDataTypeStr=boolean
  Logical Operator5 : Logic  Operator=OR  AllPortsSameDT=off  OutDataTypeStr=boolean
  Relational Operator6 : RelationalOperator  Operator===  OutDataTypeStr=boolean  RndMeth=Simplest
  Relational Operator7 : RelationalOperator  Operator===  OutDataTypeStr=boolean  RndMeth=Simplest
  Relational Operator8 : RelationalOperator  Operator===  OutDataTypeStr=boolean  RndMeth=Simplest
  Switch : Switch  Criteria=u2 ~= 0
  CrCtl_stSub_raw : Outport
  wires:
  Relational Operator8/1 -> Logical Operator4/2
  Logical Operator5/1 -> Logical Operator4/1
  Constant10/1 -> Switch/1
  CrCtl_stSub/1 -> Relational Operator8/1, Switch/3
  Switch/1 -> CrCtl_stSub_raw/1
  Logical Operator4/1 -> Switch/2
  CrCtl_st/1 -> Relational Operator6/1, Relational Operator7/1
  Constant8/1 -> Relational Operator7/2
  CrCtl_stEna_mp/1 -> Logical Operator4/3
  Constant7/1 -> Relational Operator6/2
  Relational Operator7/1 -> Logical Operator5/2
  Relational Operator6/1 -> Logical Operator5/1
  Constant9/1 -> Relational Operator8/2

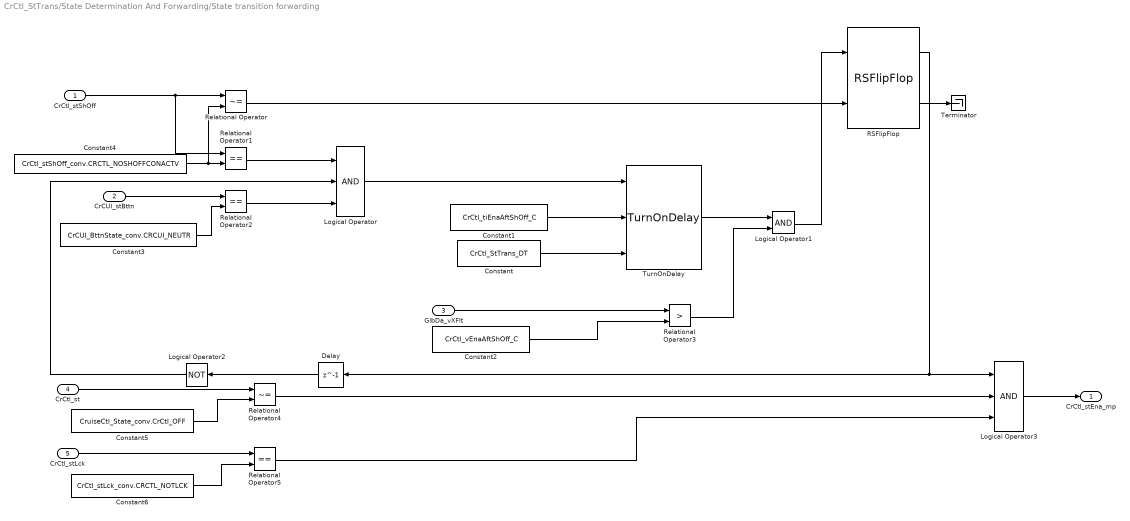
== system CrCtl_StTrans/State Determination And Forwarding/State transition forwarding ==
  CrCtl_stShOff : Inport
  CrCUI_stBttn : Inport  Port=2
  GlbDa_vXFlt : Inport  Port=3
  CrCtl_st : Inport  Port=4
  CrCtl_stLck : Inport  Port=5
  Constant : Constant  Value=CrCtl_StTrans_DT
  Constant1 : Constant  Value=CrCtl_tiEnaAftShOff_C
  Constant2 : Constant  Value=CrCtl_vEnaAftShOff_C
  Constant3 : Constant  Value=CrCUI_BttnState_conv.CRCUI_NEUTR
  Constant4 : Constant  Value=CrCtl_stShOff_conv.CRCTL_NOSHOFFCONACTV
  Constant5 : Constant  Value=CruiseCtl_State_conv.CrCtl_OFF
  Constant6 : Constant  Value=CrCtl_stLck_conv.CRCTL_NOTLCK
  Delay : Delay  DelayLength=1  InputProcessing=Inherited
  Logical Operator : Logic  Inputs=3  AllPortsSameDT=off  OutDataTypeStr=boolean
  Logical Operator1 : Logic  AllPortsSameDT=off  OutDataTypeStr=boolean
  Logical Operator2 : Logic  Operator=NOT  AllPortsSameDT=off  OutDataTypeStr=boolean
  Logical Operator3 : Logic  Inputs=3  AllPortsSameDT=off  OutDataTypeStr=boolean
  RSFlipFlop : CXLib/RSFlipFlop
  Relational Operator : RelationalOperator  Operator=~=  OutDataTypeStr=boolean  RndMeth=Simplest
  Relational Operator1 : RelationalOperator  Operator===  OutDataTypeStr=boolean  RndMeth=Simplest
  Relational Operator2 : RelationalOperator  Operator===  OutDataTypeStr=boolean  RndMeth=Simplest
  Relational Operator3 : RelationalOperator  Operator=>  OutDataTypeStr=boolean  RndMeth=Simplest
  Relational Operator4 : RelationalOperator  Operator=~=  OutDataTypeStr=boolean  RndMeth=Simplest
  Relational Operator5 : RelationalOperator  Operator===  OutDataTypeStr=boolean  RndMeth=Simplest
  Terminator : Terminator
  TurnOnDelay : CXLib/TurnOnDelay
  CrCtl_stEna_mp : Outport
  wires:
  Relational Operator3/1 -> Logical Operator1/2
  RSFlipFlop/2 -> Terminator/1
  GlbDa_vXFlt/1 -> Relational Operator3/1
  Relational Operator4/1 -> Logical Operator3/2
  Relational Operator5/1 -> Logical Operator3/3
  Constant6/1 -> Relational Operator5/2
  Relational Operator1/1 -> Logical Operator/1
  Logical Operator/1 -> TurnOnDelay/1
  Relational Operator/1 -> RSFlipFlop/2
  CrCtl_stShOff/1 -> Relational Operator1/1, Relational Operator/1
  CrCUI_stBttn/1 -> Relational Operator2/1
  Constant3/1 -> Relational Operator2/2
  CrCtl_stLck/1 -> Relational Operator5/1
  Constant4/1 -> Relational Operator/2, Relational Operator1/2
  Constant/1 -> TurnOnDelay/3
  Constant1/1 -> TurnOnDelay/2
  Logical Operator3/1 -> CrCtl_stEna_mp/1
  RSFlipFlop/1 -> Logical Operator3/1, Delay/1
  Constant5/1 -> Relational Operator4/2
  Logical Operator1/1 -> RSFlipFlop/1
  Logical Operator2/1 -> Logical Operator/2
  Constant2/1 -> Relational Operator3/2
  TurnOnDelay/1 -> Logical Operator1/1
  CrCtl_st/1 -> Relational Operator4/1
  Relational Operator2/1 -> Logical Operator/3
  Delay/1 -> Logical Operator2/1
